simulink model "Fig241"  (R2014a)
settings: Solver=FixedStepDiscrete  StartTime=0.0  StopTime=5.2488  FixedStep=2e-5  RelTol=1e-3
libraries: commutil2 x1, commrandsrc2 x1
settings Model: Creator=Dennis Silage  LastModifiedBy=Silage
settings DataIOCC: SignalLoggingSaveFormat=ModelDataLogs
settings OptimizationCC: ExpressionDepthLimit=2147483647  InitFltsAndDblsToZero=on
settings DebuggingCC: UnderspecifiedInitializationDetection=Classic  FcnCallInpInsideContextMsg=UseLocalSettings  StateNameClashWarn=warning
settings GRTTargetCC: CombineOutputUpdateFcns=off  GRTInterface=on

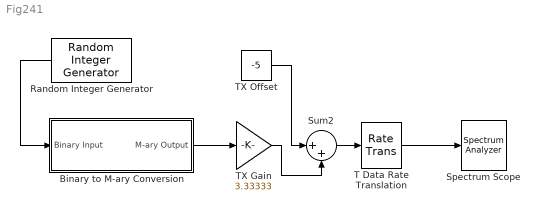
== system Fig241 ==
  Binary to M-ary Conversion : Subsystem
  Random Integer Generator : commrandsrc2/Random Integer Generator  mul=2  seed=randseed  Ts=1e-3  frameBased=off  sampPerFrame=1  orient=off  outDataType=double
  Spectrum Scope : SpectrumAnalyzer
  Sum2 : Sum  Inputs=|++
  T Data Rate Translation : RateTransition  OutPortSampleTime=2e-5
  TX Gain : Gain  Gain=3.33333
  TX Offset : Constant  Value=-5
  wires:
  TX Gain/1 -> Sum2/2
  TX Offset/1 -> Sum2/1
  Sum2/1 -> T Data Rate Translation/1
  Random Integer Generator/1 -> Binary to M-ary Conversion/1(Binary Input)
  Binary to M-ary Conversion/1("M-ary Output ") -> TX Gain/1
  T Data Rate Translation/1 -> Spectrum Scope/1

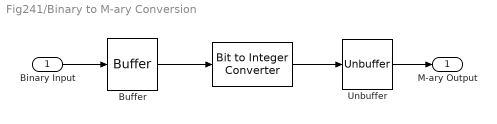
== system Fig241/Binary to M-ary Conversion ==
  Binary Input : Inport
  " " : commutil2/Bit to Integer Converter  nbits=2  bitOrder=MSB first  signedOutputValues=Unsigned  outDtype=Inherit via internal rule  outDtypeSigned=Inherit via internal rule
  Buffer : Buffer  N=2  TreatMby1Signals=One channel
  Unbuffer : Unbuffer  SampleBasedProcessing=Same as frame based
  "M-ary Output " : Outport
  wires:
  Binary Input/1 -> Buffer/1
  Buffer/1 -> " "/1
  " "/1 -> Unbuffer/1
  Unbuffer/1 -> "M-ary Output "/1
